simulink model "VB_RIFKF_UWB_INS25"  (R2023a)
settings: Solver=FixedStepAuto  StartTime=0.0  StopTime=500  FixedStep=0.01  RelTol=1e-3
InitFcn:
  | resilient_initNavigation1216;
  | init_param;
  | param_bias;
undefined symbols (not defined in the file or in its folder): dt, g0, gam0_rad, ISUS_flag, lp_GPS_sample_time, lp_Lidar_knoise, lp_Lidar_max, lp_Lidar_min, lp_Lidar_sample_time, lp_Lidar_seed, lp_UWB_knoise, lp_UWB_sample_time, lp_UWB_seed, lp_UWB_XY_max, lp_UWB_XY_min, magnitude, p, P0, P0_RIEKF, param, pd0, pe0, phi0_rad, pn0, psi, psi0_rad, state_dim, vd0, ve0, vn0
libraries: simulink_extras x108, simulink x89, dspstat3 x74, sharedtransform x61, matrix_library x11, sharedTrackingLibrary x8, aerolibconvert2 x5, aerolibtransform2 x5, dspfactors x3
(part 1 of 29)
settings Model: PacingRate=0.089000  Creator=Ye Xiaoyu  LastModifiedBy=18296
settings DataIOCC: SaveFormat=Structure
settings DebuggingCC: ParameterPrecisionLossMsg=none

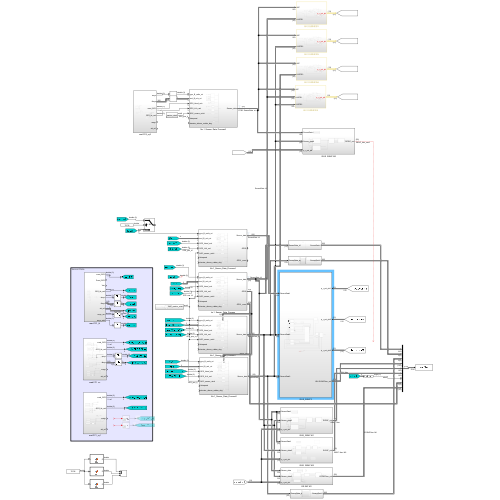
[thumbnail: Simulink's stored preview of the top-level diagram]
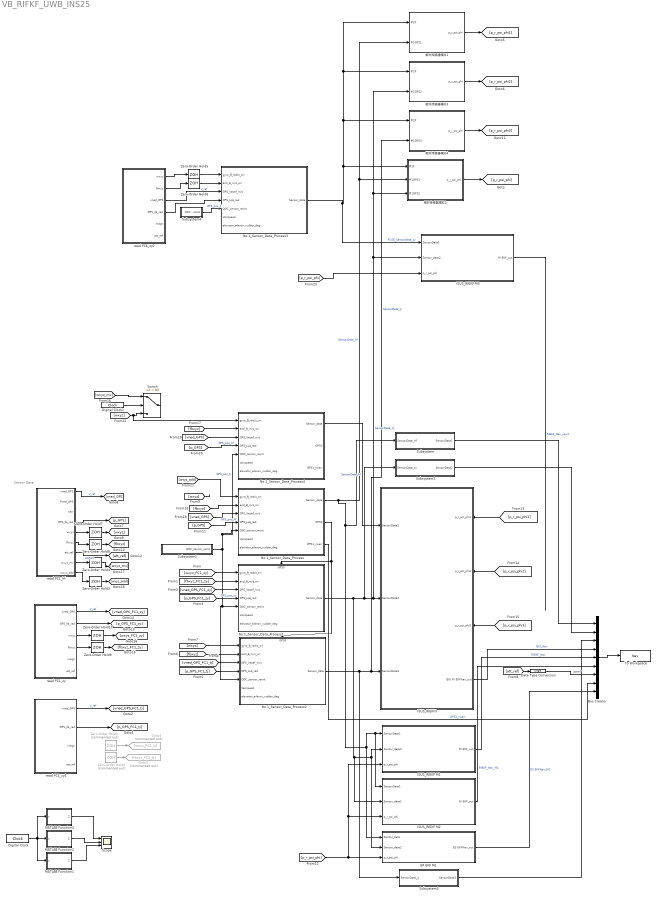
== system VB_RIFKF_UWB_INS25 ==
  note: Sensor Data
  Bus Creator : BusCreator  Inputs=9
  Data Type Conversion : DataTypeConversion  OutDataTypeStr=single  SaturateOnIntegerOverflow=off  RndMeth=Floor
  Digital Clock : DigitalClock  SampleTime=0.01
  Digital Clock1 : DigitalClock  SampleTime=0.01
  ER EKF M1 : Subsystem
  Goto3 : Goto  Commented=on  GotoTag=fbxyz_FC1_tj
  Goto4 : Goto  Commented=on  GotoTag=wxyz_FC1_tj
  ISUS_RIEKF M1 : Subsystem
  ISUS_RIEKF M2 : Subsystem
  ISUS_RIEKF M3 : Subsystem
  ISUS_RIEKF3 : Subsystem
      settings: PortSchema="{\"entries\":[{\"content\":{\"sides\":[{\"content\":{\"connectorIds\":[\"In1\",\"In2\",\"In3\"]},\"type\":\"ConnectorPlacement.EquallySpacedRectSide\",\"uuid\":\"2bcd161f-da55-4ee1-9ea8-951282ac87a0\"},{\"content\":{\"connectorIds\":[\"In4\",\"In5\",\"In6\",\"Out1\"],\"side\":\"RIGHT\"},\"type\":\"ConnectorPlacement.EquallySpacedRectSide\",\"uuid\":\"1132c6d7-5262-4ef0-a9d0-f977b200d157\"},{\"content\":{\"side\":\"TOP\"},\"type\":\"ConnectorPlacement.EquallySpacedRectSide\",\"uuid\":\"5bcb3a10-5be6-4cd2-9d61-0144f4936936\"}]},\"type\":\"ConnectorPlacement.EquallySpacedConnector\",\"uuid\":\"76638c5d-0c18-4b86-9384-f3a5e1322473\"}],\"packageUris\":[\"http://schema.mathworks.com/mf0/Connector/R2020b\"],\"version\":\"1.0\"}"
  MATLAB Function1 : MATLAB Function  TreatAsAtomicUnit=on
  MATLAB Function2 : MATLAB Function  TreatAsAtomicUnit=on
  MATLAB Function3 : MATLAB Function  TreatAsAtomicUnit=on
  No.1_Sensor_Data_Process : Subsystem
  No.1_Sensor_Data_Process1 : Subsystem
      settings: PortSchema="{\"entries\":[{\"content\":{\"sides\":[{\"content\":{\"connectorIds\":[\"In1\",\"In2\",\"In3\",\"In4\",\"In5\",\"In6\",\"In7\"]},\"type\":\"ConnectorPlacement.EquallySpacedRectSide\",\"uuid\":\"9a461442-5a4c-405b-8781-00f946dfe93c\"},{\"content\":{\"connectorIds\":[\"Out1\"],\"side\":\"RIGHT\"},\"type\":\"ConnectorPlacement.EquallySpacedRectSide\",\"uuid\":\"70ca8ff8-5980-4d24-aa39-0c8562a9d1d9\"},{\"content\":{\"connectorIds\":[\"In8\"],\"side\":\"TOP\"},\"type\":\"ConnectorPlacement.EquallySpacedRectSide\",\"uuid\":\"b1ebbd88-9925-4860-b235-fb3cc0770858\"}]},\"type\":\"ConnectorPlacement.EquallySpacedConnector\",\"uuid\":\"3dd6f087-9fad-422a-adf7-c884c798750f\"}],\"packageUris\":[\"http://schema.mathworks.com/mf0/Connector/R2020b\"],\"version\":\"1.0\"}"
  No.1_Sensor_Data_Process2 : Subsystem
      settings: PortSchema="{\"entries\":[{\"content\":{\"sides\":[{\"content\":{\"connectorIds\":[\"In1\",\"In2\",\"In3\",\"In4\",\"In5\",\"In6\",\"In7\"]},\"type\":\"ConnectorPlacement.EquallySpacedRectSide\",\"uuid\":\"9a461442-5a4c-405b-8781-00f946dfe93c\"},{\"content\":{\"connectorIds\":[\"Out1\"],\"side\":\"RIGHT\"},\"type\":\"ConnectorPlacement.EquallySpacedRectSide\",\"uuid\":\"70ca8ff8-5980-4d24-aa39-0c8562a9d1d9\"},{\"content\":{\"connectorIds\":[\"In8\"],\"side\":\"TOP\"},\"type\":\"ConnectorPlacement.EquallySpacedRectSide\",\"uuid\":\"b1ebbd88-9925-4860-b235-fb3cc0770858\"}]},\"type\":\"ConnectorPlacement.EquallySpacedConnector\",\"uuid\":\"3dd6f087-9fad-422a-adf7-c884c798750f\"}],\"packageUris\":[\"http://schema.mathworks.com/mf0/Connector/R2020b\"],\"version\":\"1.0\"}"
  No.1_Sensor_Data_Process3 : Subsystem
  No.1_Sensor_Data_Process4 : Subsystem
  Scope : Scope  NumInputPorts=3
  Subsystem : Subsystem
  Subsystem1 : Subsystem
  Subsystem2 : Subsystem
  Subsystem3 : Subsystem
  Subsystem4 : Subsystem
  Switch : Switch  Criteria=u2 > Threshold  Threshold=80  SaturateOnIntegerOverflow=off  InputSameDT=off
  To Workspace : ToWorkspace  VariableName=Nav  SaveFormat=Timeseries  SampleTime=0.01
  Zero-Order Hold1 : ZeroOrderHold  Commented=on  SampleTime=dt
  Zero-Order Hold{3..10} (8 alike) : ZeroOrderHold  SampleTime=dt
  Zero-Order Hold2 : ZeroOrderHold  Commented=on  SampleTime=dt
  read FC1_hf : Subsystem
  read FC1_zy : Subsystem
  read FC1_zy1 : Subsystem
  read FC6_zy2 : Subsystem
  相对传感器模拟1 : Subsystem
  相对传感器模拟2 : Subsystem
  相对传感器模拟3 : Subsystem
  相对传感器模拟4 : Subsystem
  wires:
  read FC1_hf/1(vned_GPS) -> [vned_GPS]  "V_ref"
  read FC1_hf/6(fbxyz) -> Zero-Order Hold8/1
  read FC1_hf/5(wxyz) -> Zero-Order Hold7/1
  read FC1_hf/7(att_ref) -> [att_ref]  "att_ref"
  read FC1_zy/2(GPS_lla_rad) -> [p_GPS_FC1_zy]
  read FC1_zy/1(vned_GPS) -> [vned_GPS_FC1_zy]  "V_ref"
  read FC1_hf/4(GPS_lla_rad) -> [p_GPS]
  Zero-Order Hold10/1 -> [wxyz_FC1_zy]
  Zero-Order Hold9/1 -> [fbxyz_FC1_zy]
  read FC1_zy/3(wxyz) -> Zero-Order Hold10/1
  read FC1_zy/4(fbxyz) -> Zero-Order Hold9/1
  Zero-Order Hold7/1 -> [wxyz]
  Zero-Order Hold8/1 -> [fbxyz]
  [fbxyz] -> No.1_Sensor_Data_Process/2(accl_B_m/s_ori)
  Subsystem1/1(QGC_sensor_reinit) -> No.1_Sensor_Data_Process4/5(QGC_sensor_reinit), No.1_Sensor_Data_Process/5(QGC_sensor_reinit), No.1_Sensor_Data_Process1/5(QGC_sensor_reinit), No.1_Sensor_Data_Process2/5(QGC_sensor_reinit)  "GPS_pos_tj"
  [wxyz] -> ?
  No.1_Sensor_Data_Process1/1(Sensor_data) -> ISUS_RIEKF3/2(SensorData2), 相对传感器模拟3/2(#1GPS2), 相对传感器模拟2/3(#1GPS2), ISUS_RIEKF M3/2(Sensor_data2), Subsystem2/1(SensorData_zy), ISUS_RIEKF M2/2(Sensor_data2), ER EKF M1/2(Sensor_data2), ISUS_RIEKF M1/2(Sensor_data2)  "SensorData_zy"
  [wxyz_FC1_zy] -> No.1_Sensor_Data_Process1/1(gyro_B_rad/s_ori)
  [fbxyz_FC1_zy] -> No.1_Sensor_Data_Process1/2(accl_B_m/s_ori)
  [vned_GPS] -> No.1_Sensor_Data_Process/3(GPS_Vecef_m/s)
  [p_GPS] -> No.1_Sensor_Data_Process/4(GPS_LLA_rad)  "GPS_pos_hf"
  [vned_GPS_FC1_zy] -> No.1_Sensor_Data_Process1/3(GPS_Vecef_m/s)
  [p_GPS_FC1_zy] -> No.1_Sensor_Data_Process1/4(GPS_LLA_rad)  "GPS_pos_zy"
  ? -> Zero-Order Hold2/1
  ? -> Zero-Order Hold1/1
  Zero-Order Hold2/1 -> Goto3/1
  Zero-Order Hold1/1 -> Goto4/1
  read FC1_zy1/1(vned_GPS) -> [vned_GPS_FC1_tj]  "V_ref"
  read FC1_zy1/2(GPS_lla_rad) -> [p_GPS_FC1_tj]
  [fbxyz] -> No.1_Sensor_Data_Process2/2(accl_B_m/s_ori)
  [wxyz] -> No.1_Sensor_Data_Process2/1(gyro_B_rad/s_ori)
  [vned_GPS_FC1_tj] -> No.1_Sensor_Data_Process2/3(GPS_Vecef_m/s)
  [p_GPS_FC1_tj] -> No.1_Sensor_Data_Process2/4(GPS_LLA_rad)
  No.1_Sensor_Data_Process2/1(Sensor_data) -> Subsystem3/1(SensorData_tj), ISUS_RIEKF3/3(SensorData3), 相对传感器模拟4/2(#1GPS3)  "SensorData_tj"
  ISUS_RIEKF3/1(ISIU RI EKFNav_out) -> Bus Creator/4  "ISIU_Nav"
  ISUS_RIEKF M1/1(RI EKF_out) -> Bus Creator/5  "RIEKF_Nav"
  Bus Creator/1 -> To Workspace/1
  Subsystem/1(SensorData1) -> Bus Creator/1
  Subsystem2/1(SensorData2) -> Bus Creator/2
  Subsystem3/1(SensorData3) -> Bus Creator/3
  [att_ref] -> Data Type Conversion/1
  Data Type Conversion/1 -> Bus Creator/7  "attref"
  No.1_Sensor_Data_Process/2(GPS0) -> No.1_Sensor_Data_Process2/8(GPS0), No.1_Sensor_Data_Process1/8(GPS0)
  No.1_Sensor_Data_Process/3(GPS1_noerr) -> Bus Creator/8  "GPS1_noerr"
  ISUS_RIEKF M2/1(RI EKF_out) -> Bus Creator/6  "RIEKF_Nav_M2"
  ER EKF M1/1(ES EKFNav_out) -> Bus Creator/9  "ES EKFNav_M1"
  Digital Clock/1 -> MATLAB Function3/1(t), MATLAB Function1/1(t), MATLAB Function2/1(t)
  MATLAB Function2/1(Z) -> Scope/2
  MATLAB Function1/1(Z) -> Scope/3
  MATLAB Function3/1(Z) -> Scope/1
  read FC6_zy2/4(GPS_lla_rad) -> No.1_Sensor_Data_Process3/4(GPS_LLA_rad)
  read FC6_zy2/3(vned_GPS) -> No.1_Sensor_Data_Process3/3(GPS_Vecef_m/s)  "V_ref"
  Subsystem4/1(QGC_sensor_reinit) -> No.1_Sensor_Data_Process3/5(QGC_sensor_reinit)  "GPS_pos_tj"
  No.1_Sensor_Data_Process3/1(Sensor_data) -> ISUS_RIEKF M3/1(SensorData1), 相对传感器模拟1/1(#2P), 相对传感器模拟3/1(#2P), 相对传感器模拟4/1(#2P), 相对传感器模拟2/1(#2P)  "FCS6_SensorData_zy"
  No.1_Sensor_Data_Process/1(Sensor_data) -> ER EKF M1/1(Sensor_data), ISUS_RIEKF M1/1(SensorData1), ISUS_RIEKF M2/1(SensorData1), Subsystem/1(SensorData_hf), 相对传感器模拟1/2(#1GPS1), 相对传感器模拟2/2(#1GPS1)  "SensorData_hf"
  相对传感器模拟2/1(p_r_psi_phi) -> [p_r_psi_phi]
  [p_r_psi_phi] -> ISUS_RIEKF M1/3(p_r_psi_phi), ISUS_RIEKF M2/3(p_r_psi_phi), ER EKF M1/3(p_r_psi_phi)
  相对传感器模拟1/1(p_r_psi_phi) -> [p_r_psi_phi1]
  相对传感器模拟3/1(p_r_psi_phi) -> [p_r_psi_phi2]
  相对传感器模拟4/1(p_r_psi_phi) -> [p_r_psi_phi3]
  [p_r_psi_phi1] -> ISUS_RIEKF3/4(p_r_psi_phi1)
  [p_r_psi_phi2] -> ISUS_RIEKF3/5(p_r_psi_phi2)
  [p_r_psi_phi3] -> ISUS_RIEKF3/6(p_r_psi_phi3)
  read FC1_hf/9(wxyz_add) -> Zero-Order Hold3/1
  read FC1_hf/8(wxyz_mv) -> Zero-Order Hold4/1
  Zero-Order Hold4/1 -> [wxyz_mv]
  Zero-Order Hold3/1 -> [wxyz_add]
  [wxyz_mv] -> Switch/1
  [fbxyz] -> No.1_Sensor_Data_Process4/2(accl_B_m/s_ori)
  [vned_GPS] -> No.1_Sensor_Data_Process4/3(GPS_Vecef_m/s)
  [p_GPS] -> No.1_Sensor_Data_Process4/4(GPS_LLA_rad)  "GPS_pos_hf"
  No.1_Sensor_Data_Process4/1(Sensor_data) -> ISUS_RIEKF3/1(SensorData1)  "SensorData_hf"
  [wxyz_add] -> No.1_Sensor_Data_Process/1(gyro_B_rad/s_ori)
  Digital Clock1/1 -> Switch/2
  [wxyz] -> No.1_Sensor_Data_Process4/1(gyro_B_rad/s_ori), Switch/3
  [p_r_psi_phi] -> ISUS_RIEKF M3/3(p_r_psi_phi)
  ISUS_RIEKF M3/1(RI EKF_out) -> ?  "RIEKF_Nav_uav2"
  read FC6_zy2/2(fbxyz) -> Zero-Order Hold6/1
  read FC6_zy2/1(wxyz) -> Zero-Order Hold5/1
  Zero-Order Hold5/1 -> No.1_Sensor_Data_Process3/1(gyro_B_rad/s_ori)
  Zero-Order Hold6/1 -> No.1_Sensor_Data_Process3/2(accl_B_m/s_ori)

== system VB_RIFKF_UWB_INS25/ER EKF M1 ==
  Sensor_data : Inport
  Sensor_data2 : Inport  Port=2
  p_r_psi_phi : Inport  Port=3
  Bus_Constructor : Subsystem
  Bus_Constructor2 : Subsystem
  Data Store Memory : DataStoreMemory  DataStoreName=feedback_flag_18dim  WriteAfterWriteMsg=warning  ShowAdditionalParam=off
  Data Store Memory1 : DataStoreMemory  DataStoreName=GPS_enable  WriteAfterWriteMsg=warning  ShowAdditionalParam=off
  Data Store Read : DataStoreRead  DataStoreName=GPS_enable  IndexOptions=Index vector (dialog)  Indices=1  OutputSizes=1
  Error State Kalman Filter : Subsystem
  INS propogation : Subsystem
  Sensor_data1 : InportShadow
  ES EKFNav_out : Outport
  wires:
  Sensor_data/1 -> INS propogation/1(Sensor_data)
  Error State Kalman Filter/1(delta_state) -> INS propogation/3(delta_state)
  Error State Kalman Filter/2(Measuemrnt Enable Flag) -> INS propogation/2(Measuemrnt Enable Flag)
  INS propogation/1(INSstate) -> Bus_Constructor/1(INSstate), Error State Kalman Filter/2(INS state)
  Sensor_data1/1 -> Error State Kalman Filter/1(Sensor_data)
  Bus_Constructor/1(TranslationData) -> Bus_Constructor2/1(TranlationData)
  Bus_Constructor/2(RotationData) -> Bus_Constructor2/2(RotationData)
  Bus_Constructor/3(INSbiasData) -> Bus_Constructor2/3(INSbiasData)
  Bus_Constructor2/1(RI EKFNav_out) -> ES EKFNav_out/1  "RI EKF_out"
  Sensor_data2/1 -> Error State Kalman Filter/3(Sensor_data2)
  p_r_psi_phi/1 -> Error State Kalman Filter/4(p_r_psi_phi)

== system VB_RIFKF_UWB_INS25/ISUS_RIEKF M1 ==
  SensorData1 : Inport
  Sensor_data2 : Inport  Port=2
  p_r_psi_phi : Inport  Port=3
  Bus Selector : BusSelector  OutputSignals=delta_state
  Bus_Constructor : Subsystem
  Bus_Constructor2 : Subsystem
  Data Store Memory : DataStoreMemory  DataStoreName=feedback_flag_18dim_RIEKF  WriteAfterWriteMsg=warning  ShowAdditionalParam=off
  Data Store Memory1 : DataStoreMemory  DataStoreName=GPS_enable_RIEKF  WriteAfterWriteMsg=warning  ShowAdditionalParam=off
  Error State Kalman Filter M1 : Subsystem
      settings: PortSchema="{\"entries\":[{\"content\":{\"sides\":[{\"content\":{\"connectorIds\":[\"In1\",\"In2\"]},\"type\":\"ConnectorPlacement.EquallySpacedRectSide\",\"uuid\":\"06174571-c694-4df4-9d5d-6f87fae6fca4\"},{\"content\":{\"connectorIds\":[\"Out1\",\"In3\",\"Out2\",\"In4\"],\"side\":\"RIGHT\"},\"type\":\"ConnectorPlacement.EquallySpacedRectSide\",\"uuid\":\"968b9d6c-6269-4201-a494-e936bbf59a60\"},{\"content\":{\"side\":\"TOP\"},\"type\":\"ConnectorPlacement.EquallySpacedRectSide\",\"uuid\":\"42ff394f-5689-4ff8-9152-3bae82104e67\"}]},\"type\":\"ConnectorPlacement.EquallySpacedConnector\",\"uuid\":\"445a129c-1b79-435d-8e29-ecc9e3655f53\"}],\"packageUris\":[\"http://schema.mathworks.com/mf0/Connector/R2020b\"],\"version\":\"1.0\"}"
  INS propogation : Subsystem
  Sensor_data1 : InportShadow
  RI EKF_out : Outport
  wires:
  Bus_Constructor2/1(RI EKFNav_out) -> RI EKF_out/1  "RI EKF_out"
  Bus_Constructor/4(GNSS enable flag) -> Bus_Constructor2/4(GNSS enable flag)
  Bus_Constructor/3(INSbiasData) -> Bus_Constructor2/3(INSbiasData)  "INSbiasData"
  Bus_Constructor/2(RotationData) -> Bus_Constructor2/2(RotationData)  "RotationData"
  Bus_Constructor/1(TranslationData) -> Bus_Constructor2/1(TranlationData)  "TranslationData"
  Error State Kalman Filter M1/2(EKFstate_M1) -> Bus Selector/1
  SensorData1/1 -> INS propogation/1(Sensor_data)
  Error State Kalman Filter M1/1(Measuemrnt Enable Flag) -> INS propogation/2(Measuemrnt Enable Flag)
  INS propogation/1(INSstate) -> Bus_Constructor/1(INSstate), Error State Kalman Filter M1/2(INS state)
  Sensor_data1/1 -> Error State Kalman Filter M1/1(Sensor_data)
  Bus Selector/1 -> INS propogation/3(delta_state)  "<delta_state>"
  Sensor_data2/1 -> Error State Kalman Filter M1/3(Sensor_data2)
  p_r_psi_phi/1 -> Error State Kalman Filter M1/4(p_r_psi_phi1)

== system VB_RIFKF_UWB_INS25/ISUS_RIEKF M2 ==
  SensorData1 : Inport
  Sensor_data2 : Inport  Port=2
  p_r_psi_phi : Inport  Port=3
  Bus Selector : BusSelector  OutputSignals=delta_state
  Bus_Constructor : Subsystem
  Bus_Constructor2 : Subsystem
  Data Store Memory : DataStoreMemory  DataStoreName=feedback_flag_18dim_RIEKF  WriteAfterWriteMsg=warning  ShowAdditionalParam=off
  Data Store Memory1 : DataStoreMemory  DataStoreName=GPS_enable_RIEKF  WriteAfterWriteMsg=warning  ShowAdditionalParam=off
  Error State Kalman Filter M1 : Subsystem
      settings: PortSchema="{\"entries\":[{\"content\":{\"sides\":[{\"content\":{\"connectorIds\":[\"In1\",\"In2\"]},\"type\":\"ConnectorPlacement.EquallySpacedRectSide\",\"uuid\":\"06174571-c694-4df4-9d5d-6f87fae6fca4\"},{\"content\":{\"connectorIds\":[\"Out1\",\"In3\",\"Out2\",\"In4\"],\"side\":\"RIGHT\"},\"type\":\"ConnectorPlacement.EquallySpacedRectSide\",\"uuid\":\"968b9d6c-6269-4201-a494-e936bbf59a60\"},{\"content\":{\"side\":\"TOP\"},\"type\":\"ConnectorPlacement.EquallySpacedRectSide\",\"uuid\":\"42ff394f-5689-4ff8-9152-3bae82104e67\"}]},\"type\":\"ConnectorPlacement.EquallySpacedConnector\",\"uuid\":\"445a129c-1b79-435d-8e29-ecc9e3655f53\"}],\"packageUris\":[\"http://schema.mathworks.com/mf0/Connector/R2020b\"],\"version\":\"1.0\"}"
  Error State Kalman Filter M3 : Subsystem  Commented=on
  Error State Kalman Filter M4 : Subsystem  Commented=on
      settings: PortSchema="{\"entries\":[{\"content\":{\"sides\":[{\"content\":{\"connectorIds\":[\"In1\",\"In2\"]},\"type\":\"ConnectorPlacement.EquallySpacedRectSide\",\"uuid\":\"06174571-c694-4df4-9d5d-6f87fae6fca4\"},{\"content\":{\"connectorIds\":[\"Out1\",\"In3\",\"Out2\",\"In4\"],\"side\":\"RIGHT\"},\"type\":\"ConnectorPlacement.EquallySpacedRectSide\",\"uuid\":\"968b9d6c-6269-4201-a494-e936bbf59a60\"},{\"content\":{\"side\":\"TOP\"},\"type\":\"ConnectorPlacement.EquallySpacedRectSide\",\"uuid\":\"42ff394f-5689-4ff8-9152-3bae82104e67\"}]},\"type\":\"ConnectorPlacement.EquallySpacedConnector\",\"uuid\":\"445a129c-1b79-435d-8e29-ecc9e3655f53\"}],\"packageUris\":[\"http://schema.mathworks.com/mf0/Connector/R2020b\"],\"version\":\"1.0\"}"
  INS propogation1 : Subsystem
  INS propogation2 : Subsystem  Commented=on
  Sensor_data1 : InportShadow
  RI EKF_out : Outport
  wires:
  Bus Selector/1 -> INS propogation1/3(delta_state)  "<delta_state>"
  Sensor_data1/1 -> Error State Kalman Filter M1/1(Sensor_data)
  INS propogation1/1(INSstate) -> Error State Kalman Filter M1/2(INS state), Bus_Constructor/1(INSstate)
  SensorData1/1 -> INS propogation1/1(Sensor_data)
  Error State Kalman Filter M1/2(EKFstate_M1) -> Bus Selector/1
  Bus_Constructor/1(TranslationData) -> Bus_Constructor2/1(TranlationData)  "TranslationData"
  Bus_Constructor/2(RotationData) -> Bus_Constructor2/2(RotationData)  "RotationData"
  Bus_Constructor/3(INSbiasData) -> Bus_Constructor2/3(INSbiasData)  "INSbiasData"
  Bus_Constructor/4(GNSS enable flag) -> Bus_Constructor2/4(GNSS enable flag)
  Bus_Constructor2/1(RI EKFNav_out) -> RI EKF_out/1  "RI EKF_out"
  Error State Kalman Filter M1/1(Measuemrnt Enable Flag) -> INS propogation1/2(Measuemrnt Enable Flag)
  Sensor_data2/1 -> Error State Kalman Filter M1/3(Sensor_data2)
  p_r_psi_phi/1 -> Error State Kalman Filter M1/4(p_r_psi_phi1)

== system VB_RIFKF_UWB_INS25/ISUS_RIEKF M3 ==
  SensorData1 : Inport
  Sensor_data2 : Inport  Port=2
  p_r_psi_phi : Inport  Port=3
  Bus Selector : BusSelector  OutputSignals=delta_state
  Bus_Constructor : Subsystem
  Bus_Constructor2 : Subsystem
  Data Store Memory : DataStoreMemory  DataStoreName=feedback_flag_18dim_RIEKF  WriteAfterWriteMsg=warning  ShowAdditionalParam=off
  Data Store Memory1 : DataStoreMemory  DataStoreName=GPS_enable_RIEKF  WriteAfterWriteMsg=warning  ShowAdditionalParam=off
  Error State Kalman Filter M1 : Subsystem
      settings: PortSchema="{\"entries\":[{\"content\":{\"sides\":[{\"content\":{\"connectorIds\":[\"In1\",\"In2\"]},\"type\":\"ConnectorPlacement.EquallySpacedRectSide\",\"uuid\":\"06174571-c694-4df4-9d5d-6f87fae6fca4\"},{\"content\":{\"connectorIds\":[\"Out1\",\"In3\",\"Out2\",\"In4\"],\"side\":\"RIGHT\"},\"type\":\"ConnectorPlacement.EquallySpacedRectSide\",\"uuid\":\"968b9d6c-6269-4201-a494-e936bbf59a60\"},{\"content\":{\"side\":\"TOP\"},\"type\":\"ConnectorPlacement.EquallySpacedRectSide\",\"uuid\":\"42ff394f-5689-4ff8-9152-3bae82104e67\"}]},\"type\":\"ConnectorPlacement.EquallySpacedConnector\",\"uuid\":\"445a129c-1b79-435d-8e29-ecc9e3655f53\"}],\"packageUris\":[\"http://schema.mathworks.com/mf0/Connector/R2020b\"],\"version\":\"1.0\"}"
  INS propogation : Subsystem
  Sensor_data1 : InportShadow
  RI EKF_out : Outport
  wires:
  Bus_Constructor2/1(RI EKFNav_out) -> RI EKF_out/1  "RI EKF_out"
  Bus_Constructor/4(GNSS enable flag) -> Bus_Constructor2/4(GNSS enable flag)
  Bus_Constructor/3(INSbiasData) -> Bus_Constructor2/3(INSbiasData)  "INSbiasData"
  Bus_Constructor/2(RotationData) -> Bus_Constructor2/2(RotationData)  "RotationData"
  Bus_Constructor/1(TranslationData) -> Bus_Constructor2/1(TranlationData)  "TranslationData"
  Error State Kalman Filter M1/2(EKFstate_M1) -> Bus Selector/1
  SensorData1/1 -> INS propogation/1(Sensor_data)
  Error State Kalman Filter M1/1(Measuemrnt Enable Flag) -> INS propogation/2(Measuemrnt Enable Flag)
  INS propogation/1(INSstate) -> Bus_Constructor/1(INSstate), Error State Kalman Filter M1/2(INS state)
  Sensor_data1/1 -> Error State Kalman Filter M1/1(Sensor_data)
  Bus Selector/1 -> INS propogation/3(delta_state)  "<delta_state>"
  Sensor_data2/1 -> Error State Kalman Filter M1/3(Sensor_data2)
  p_r_psi_phi/1 -> Error State Kalman Filter M1/4(p_r_psi_phi1)

== system VB_RIFKF_UWB_INS25/ISUS_RIEKF3 ==
  SensorData1 : Inport
  SensorData2 : Inport  Port=2
  SensorData3 : Inport  Port=3
  p_r_psi_phi1 : Inport  Port=4
  p_r_psi_phi2 : Inport  Port=5
  p_r_psi_phi3 : Inport  Port=6
  Bus Creator : BusCreator  Inputs=2
  Bus_Constructor : Subsystem
  Bus_Constructor2 : Subsystem
      settings: PortSchema="{\"entries\":[{\"content\":{\"sides\":[{\"content\":{\"connectorIds\":[\"In1\",\"In2\",\"In3\",\"In4\",\"In5\",\"In6\",\"In7\"]},\"type\":\"ConnectorPlacement.EquallySpacedRectSide\",\"uuid\":\"2ada5c99-a5a9-492d-97a7-10d7c05175d7\"},{\"content\":{\"connectorIds\":[\"Out1\"],\"side\":\"RIGHT\"},\"type\":\"ConnectorPlacement.EquallySpacedRectSide\",\"uuid\":\"cde580e4-aba0-41e6-ab1b-1e880cd106da\"},{\"content\":{\"side\":\"TOP\"},\"type\":\"ConnectorPlacement.EquallySpacedRectSide\",\"uuid\":\"542037bf-a2f3-4431-b2f0-0d887f8b5219\"},{\"content\":{\"connectorIds\":[\"In8\"],\"side\":\"BOTTOM\"},\"type\":\"ConnectorPlacement.EquallySpacedRectSide\",\"uuid\":\"59daa5b1-1426-4f22-83e7-df6003f21326\"}]},\"type\":\"ConnectorPlacement.EquallySpacedConnector\",\"uuid\":\"47431650-46c1-4f35-bd73-f1f710c66ac0\"}],\"packageUris\":[\"http://schema.mathworks.com/mf0/Connector/R2020b\"],\"version\":\"1.0\"}"
  Data Store Memory : DataStoreMemory  DataStoreName=feedback_flag_18dim_RIEKF  WriteAfterWriteMsg=warning  ShowAdditionalParam=off
  Data Store Memory1 : DataStoreMemory  DataStoreName=GPS_enable_RIEKF  WriteAfterWriteMsg=warning  ShowAdditionalParam=off
  Error State Kalman Filter M1 : Subsystem
  Error State Kalman Filter M2 : Subsystem
  Error State Kalman Filter M4 : Subsystem
  Extract Diagonal1 : matrix_library/Extract Diagonal
  INS propogation : Subsystem
  INS propogation1 : Subsystem
  INS propogation2 : Subsystem
  INS propogation3 : Subsystem
  Reshape : Reshape
  Scope2 : Scope
  Sensor_data1 : InportShadow
  Subsystem : Subsystem
  Terminator : Terminator
  Terminator2 : Terminator
  ISIU RI EKFNav_out : Outport
  wires:
  Extract Diagonal1/1 -> Scope2/1  "covariance_diag"
  Subsystem/1(P_mixed_RIEKF_M1) -> Error State Kalman Filter M4/3(P_mixed_RIEKF_model1)
  Reshape/1 -> Bus Creator/2
  Bus Creator/1 -> Bus_Constructor2/8(ISIU)
  ? -> Reshape/1  "L_k"
  ? -> Bus Creator/1  "mu_k"
  Subsystem/7(X_mixed_RIEKF_M3) -> Error State Kalman Filter M2/4(X_mixed_RIEKF_M3)
  Subsystem/8(P_mixed_RIEKF_M3) -> Error State Kalman Filter M2/3(P_mixed_RIEKF_model3)
  Error State Kalman Filter M2/2(EKFstate_M3) -> Bus_Constructor2/7(EKFstate_M3), Subsystem/3(EKFstate_M3)
  Error State Kalman Filter M2/1(Measuemrnt Enable Flag) -> Terminator2/1
  SensorData3/1 -> Error State Kalman Filter M2/1(Sensor_data)
  Subsystem/6(pk_k) -> Extract Diagonal1/1
  Bus_Constructor2/1(RI EKFNav_out) -> ISIU RI EKFNav_out/1  "ISIU RI EKFNav_out"
  Bus_Constructor/4(GNSS enable flag) -> Bus_Constructor2/4(GNSS enable flag)
  Bus_Constructor/3(INSbiasData) -> Bus_Constructor2/3(INSbiasData)  "INSbiasData"
  Bus_Constructor/2(RotationData) -> Bus_Constructor2/2(RotationData)  "RotationData"
  Bus_Constructor/1(TranslationData) -> Bus_Constructor2/1(TranlationData)  "TranslationData"
  Error State Kalman Filter M4/2(EKFstate_M1) -> Bus_Constructor2/5(EKFstate_M1), Subsystem/1(EKFstate_M1)
  Subsystem/4(X_mixed_RIEKF_M2) -> Error State Kalman Filter M1/4(X_mixed_RIEKF_M2)
  Subsystem/3(P_mixed_RIEKF_M2) -> Error State Kalman Filter M1/3(P_mixed_RIEKF_model2)
  Subsystem/2(X_mixed_RIEKF_M1) -> Error State Kalman Filter M4/4(X_mixed_RIEKF_M1)
  Error State Kalman Filter M1/2(EKFstate_M2) -> Bus_Constructor2/6(EKFstate_M2), Subsystem/2(EKFstate_M2)
  Error State Kalman Filter M1/1(Measuemrnt Enable Flag) -> Terminator/1
  SensorData2/1 -> Error State Kalman Filter M1/1(Sensor_data)
  SensorData1/1 -> INS propogation/1(Sensor_data), INS propogation1/1(Sensor_data), INS propogation2/1(Sensor_data), INS propogation3/1(Sensor_data)
  Error State Kalman Filter M4/1(Measuemrnt Enable Flag) -> INS propogation3/2(Measuemrnt Enable Flag), INS propogation2/2(Measuemrnt Enable Flag), INS propogation1/2(Measuemrnt Enable Flag), INS propogation/2(Measuemrnt Enable Flag)
  Sensor_data1/1 -> Error State Kalman Filter M4/1(Sensor_data)
  Error State Kalman Filter M4/3(delta_state) -> INS propogation1/3(delta_state)
  Error State Kalman Filter M2/3(delta_state) -> INS propogation3/3(delta_state)
  Subsystem/5(xk_k) -> INS propogation/3(delta_state)
  INS propogation/1(INSstate) -> Bus_Constructor/1(INSstate)
  Error State Kalman Filter M1/3(delta_state) -> INS propogation2/3(delta_state)
  INS propogation2/1(INSstate) -> Error State Kalman Filter M1/2(INS state)
  INS propogation3/1(INSstate) -> Error State Kalman Filter M2/2(INS state)
  INS propogation1/1(INSstate) -> Error State Kalman Filter M4/2(INS state)
  p_r_psi_phi1/1 -> Error State Kalman Filter M4/5(p_r_psi_phi1)
  p_r_psi_phi2/1 -> Error State Kalman Filter M1/5(p_r_psi_phi2)
  p_r_psi_phi3/1 -> Error State Kalman Filter M2/5(p_r_psi_phi3)

== system VB_RIFKF_UWB_INS25/No.1_Sensor_Data_Process ==
  gyro_B_rad/s_ori : Inport
  accl_B_m/s_ori : Inport  Port=2
  GPS_Vecef_m/s : Inport  Port=3
  GPS_LLA_rad : Inport  Port=4
  QGC_sensor_reinit : Inport  Port=5
  Vairspeed : Inport  Port=6
  elevator_aileron_rudder_deg : Inport  Port=7
  Bus Creator : BusCreator  Inputs=8
  Constant3 : Constant
  Constant4 : Constant  Value=0.8
  Data Type Conversion{,1..3,5..6,8..11} (10 alike) : DataTypeConversion  OutDataTypeStr=single  SaturateOnIntegerOverflow=off  RndMeth=Floor
  Data Type Conversion4 : DataTypeConversion  OutDataTypeStr=uint8  SaturateOnIntegerOverflow=off  RndMeth=Floor
  Data Type Conversion7 : DataTypeConversion  OutDataTypeStr=double  SaturateOnIntegerOverflow=off  RndMeth=Floor
  GPS_Data_Process : Subsystem
  IMU_Data_Process : Subsystem
  Magn_Data_Process : Subsystem
  Mux : Mux  Inputs=3
  QGC_sensor_reinit1 : InportShadow  Port=5
  QGC_sensor_reinit2 : InportShadow  Port=5
  Subsystem : Subsystem
  TOF_Data_Process : Subsystem
  baro_Data_Process : Subsystem
  Sensor_data : Outport
  GPS0 : Outport  Port=2
  GPS1_noerr : Outport  Port=3
  wires:
  QGC_sensor_reinit2/1 -> TOF_Data_Process/2(QGC_sensor_reinit)  "QGC_sensor_reinit"
  Data Type Conversion3/1 -> baro_Data_Process/3(baro_tem)
  Data Type Conversion10/1 -> TOF_Data_Process/1(TOF_mm_ori)
  Data Type Conversion6/1 -> Magn_Data_Process/1(magn_B_guass_ori)
  Data Type Conversion5/1 -> baro_Data_Process/1(baro)
  Data Type Conversion9/1 -> GPS_Data_Process/4(hdop_GPS)
  Data Type Conversion4/1 -> GPS_Data_Process/3(GPS_fixtype)
  Data Type Conversion7/1 -> GPS_Data_Process/2(GPS_LLA_rad)
  Data Type Conversion2/1 -> GPS_Data_Process/1(GPS_Vecef_m/s)
  Data Type Conversion1/1 -> IMU_Data_Process/2(accl_B_m/s_ori)
  Data Type Conversion/1 -> IMU_Data_Process/1(gyro_B_rad/s_ori)
  TOF_Data_Process/1(TOF_Data) -> Bus Creator/5
  QGC_sensor_reinit1/1 -> Bus Creator/7  "QGC_sensor_reinit"
  Bus Creator/1 -> Sensor_data/1
  GPS_Vecef_m/s/1 -> Data Type Conversion2/1
  GPS_LLA_rad/1 -> Data Type Conversion7/1
  accl_B_m/s_ori/1 -> Data Type Conversion1/1
  Magn_Data_Process/1(MAGN_Data) -> Bus Creator/4  "MAGN_Data"
  gyro_B_rad/s_ori/1 -> Data Type Conversion/1
  baro_Data_Process/1(BARO_Data) -> Bus Creator/3  "BARO_Data"
  IMU_Data_Process/1(IMU_Data) -> Bus Creator/1  "IMU_Data"
  GPS_Data_Process/1(GPS_Data) -> Bus Creator/2  "GPS_Data"
  QGC_sensor_reinit/1 -> GPS_Data_Process/5(QGC_sensor_reinit), baro_Data_Process/2(QGC_sensor_reinit)  "QGC_sensor_reinit"
  Vairspeed/1 -> Data Type Conversion8/1  "VairspeedData"
  Data Type Conversion8/1 -> Subsystem/1(Vairspeed)
  Subsystem/1(VairspeedData) -> Bus Creator/6
  elevator_aileron_rudder_deg/1 -> Data Type Conversion11/1  "elevator_aileron_rudder_deg"
  Data Type Conversion11/1 -> Bus Creator/8  "elevator_aileron_rudder_deg"
  Constant3/1 -> Data Type Conversion4/1
  Constant4/1 -> Data Type Conversion9/1
  Mux/1 -> Data Type Conversion6/1
  GPS_Data_Process/2(GPS0) -> GPS0/1
  GPS_Data_Process/3(GPS_noerr) -> GPS1_noerr/1

== system VB_RIFKF_UWB_INS25/No.1_Sensor_Data_Process1 ==
  gyro_B_rad/s_ori : Inport
  accl_B_m/s_ori : Inport  Port=2
  GPS_Vecef_m/s : Inport  Port=3
  GPS_LLA_rad : Inport  Port=4
  QGC_sensor_reinit : Inport  Port=5
  Vairspeed : Inport  Port=6
  elevator_aileron_rudder_deg : Inport  Port=7
  GPS0 : Inport  Port=8
  Bus Creator : BusCreator  Inputs=8
  Constant3 : Constant
  Constant4 : Constant  Value=0.8
  Data Type Conversion{,1..3,5..6,8..11} (10 alike) : DataTypeConversion  OutDataTypeStr=single  SaturateOnIntegerOverflow=off  RndMeth=Floor
  Data Type Conversion4 : DataTypeConversion  OutDataTypeStr=uint8  SaturateOnIntegerOverflow=off  RndMeth=Floor
  Data Type Conversion7 : DataTypeConversion  OutDataTypeStr=double  SaturateOnIntegerOverflow=off  RndMeth=Floor
  GPS_Data_Process : Subsystem
  IMU_Data_Process : Subsystem
  Magn_Data_Process : Subsystem
  Mux : Mux  Inputs=3
  QGC_sensor_reinit1 : InportShadow  Port=5
  QGC_sensor_reinit2 : InportShadow  Port=5
  Subsystem : Subsystem
  TOF_Data_Process : Subsystem
  baro_Data_Process : Subsystem
  Sensor_data : Outport
  wires:
  Mux/1 -> Data Type Conversion6/1
  Constant4/1 -> Data Type Conversion9/1
  Constant3/1 -> Data Type Conversion4/1
  Data Type Conversion11/1 -> Bus Creator/8  "elevator_aileron_rudder_deg"
  elevator_aileron_rudder_deg/1 -> Data Type Conversion11/1  "elevator_aileron_rudder_deg"
  Subsystem/1(VairspeedData) -> Bus Creator/6
  Data Type Conversion8/1 -> Subsystem/1(Vairspeed)
  Vairspeed/1 -> Data Type Conversion8/1  "VairspeedData"
  QGC_sensor_reinit/1 -> baro_Data_Process/2(QGC_sensor_reinit), GPS_Data_Process/5(QGC_sensor_reinit)  "QGC_sensor_reinit"
  GPS_Data_Process/1(GPS_Data) -> Bus Creator/2  "GPS_Data"
  IMU_Data_Process/1(IMU_Data) -> Bus Creator/1  "IMU_Data"
  baro_Data_Process/1(BARO_Data) -> Bus Creator/3  "BARO_Data"
  gyro_B_rad/s_ori/1 -> Data Type Conversion/1
  Magn_Data_Process/1(MAGN_Data) -> Bus Creator/4  "MAGN_Data"
  accl_B_m/s_ori/1 -> Data Type Conversion1/1
  GPS_LLA_rad/1 -> Data Type Conversion7/1
  GPS_Vecef_m/s/1 -> Data Type Conversion2/1
  Bus Creator/1 -> Sensor_data/1
  QGC_sensor_reinit1/1 -> Bus Creator/7  "QGC_sensor_reinit"
  TOF_Data_Process/1(TOF_Data) -> Bus Creator/5
  Data Type Conversion/1 -> IMU_Data_Process/1(gyro_B_rad/s_ori)
  Data Type Conversion1/1 -> IMU_Data_Process/2(accl_B_m/s_ori)
  Data Type Conversion2/1 -> GPS_Data_Process/1(GPS_Vecef_m/s)
  Data Type Conversion7/1 -> GPS_Data_Process/2(GPS_LLA_rad)
  Data Type Conversion4/1 -> GPS_Data_Process/3(GPS_fixtype)
  Data Type Conversion9/1 -> GPS_Data_Process/4(hdop_GPS)
  Data Type Conversion5/1 -> baro_Data_Process/1(baro)
  Data Type Conversion6/1 -> Magn_Data_Process/1(magn_B_guass_ori)
  Data Type Conversion10/1 -> TOF_Data_Process/1(TOF_mm_ori)
  Data Type Conversion3/1 -> baro_Data_Process/3(baro_tem)
  QGC_sensor_reinit2/1 -> TOF_Data_Process/2(QGC_sensor_reinit)  "QGC_sensor_reinit"
  GPS0/1 -> GPS_Data_Process/6(GPS0)

== system VB_RIFKF_UWB_INS25/No.1_Sensor_Data_Process2 ==
  gyro_B_rad/s_ori : Inport
  accl_B_m/s_ori : Inport  Port=2
  GPS_Vecef_m/s : Inport  Port=3
  GPS_LLA_rad : Inport  Port=4
  QGC_sensor_reinit : Inport  Port=5
  Vairspeed : Inport  Port=6
  elevator_aileron_rudder_deg : Inport  Port=7
  GPS0 : Inport  Port=8
  Bus Creator : BusCreator  Inputs=8
  Constant3 : Constant
  Constant4 : Constant  Value=0.8
  Data Type Conversion{,1..3,5..6,8..11} (10 alike) : DataTypeConversion  OutDataTypeStr=single  SaturateOnIntegerOverflow=off  RndMeth=Floor
  Data Type Conversion4 : DataTypeConversion  OutDataTypeStr=uint8  SaturateOnIntegerOverflow=off  RndMeth=Floor
  Data Type Conversion7 : DataTypeConversion  OutDataTypeStr=double  SaturateOnIntegerOverflow=off  RndMeth=Floor
  GPS_Data_Process : Subsystem
  IMU_Data_Process : Subsystem
  Magn_Data_Process : Subsystem
  Mux : Mux  Inputs=3
  QGC_sensor_reinit1 : InportShadow  Port=5
  QGC_sensor_reinit2 : InportShadow  Port=5
  Subsystem : Subsystem
  TOF_Data_Process : Subsystem
  baro_Data_Process : Subsystem
  Sensor_data : Outport
  wires:
  QGC_sensor_reinit2/1 -> TOF_Data_Process/2(QGC_sensor_reinit)  "QGC_sensor_reinit"
  Data Type Conversion3/1 -> baro_Data_Process/3(baro_tem)
  Data Type Conversion10/1 -> TOF_Data_Process/1(TOF_mm_ori)
  Data Type Conversion6/1 -> Magn_Data_Process/1(magn_B_guass_ori)
  Data Type Conversion5/1 -> baro_Data_Process/1(baro)
  Data Type Conversion9/1 -> GPS_Data_Process/4(hdop_GPS)
  Data Type Conversion4/1 -> GPS_Data_Process/3(GPS_fixtype)
  Data Type Conversion7/1 -> GPS_Data_Process/2(GPS_LLA_rad)
  Data Type Conversion2/1 -> GPS_Data_Process/1(GPS_Vecef_m/s)
  Data Type Conversion1/1 -> IMU_Data_Process/2(accl_B_m/s_ori)
  Data Type Conversion/1 -> IMU_Data_Process/1(gyro_B_rad/s_ori)
  TOF_Data_Process/1(TOF_Data) -> Bus Creator/5
  QGC_sensor_reinit1/1 -> Bus Creator/7  "QGC_sensor_reinit"
  Bus Creator/1 -> Sensor_data/1
  GPS_Vecef_m/s/1 -> Data Type Conversion2/1
  GPS_LLA_rad/1 -> Data Type Conversion7/1
  accl_B_m/s_ori/1 -> Data Type Conversion1/1
  Magn_Data_Process/1(MAGN_Data) -> Bus Creator/4  "MAGN_Data"
  gyro_B_rad/s_ori/1 -> Data Type Conversion/1
  baro_Data_Process/1(BARO_Data) -> Bus Creator/3  "BARO_Data"
  IMU_Data_Process/1(IMU_Data) -> Bus Creator/1  "IMU_Data"
  GPS_Data_Process/1(GPS_Data) -> Bus Creator/2  "GPS_Data"
  QGC_sensor_reinit/1 -> GPS_Data_Process/5(QGC_sensor_reinit), baro_Data_Process/2(QGC_sensor_reinit)  "QGC_sensor_reinit"
  Vairspeed/1 -> Data Type Conversion8/1  "VairspeedData"
  Data Type Conversion8/1 -> Subsystem/1(Vairspeed)
  Subsystem/1(VairspeedData) -> Bus Creator/6
  elevator_aileron_rudder_deg/1 -> Data Type Conversion11/1  "elevator_aileron_rudder_deg"
  Data Type Conversion11/1 -> Bus Creator/8  "elevator_aileron_rudder_deg"
  Constant3/1 -> Data Type Conversion4/1
  Constant4/1 -> Data Type Conversion9/1
  Mux/1 -> Data Type Conversion6/1
  GPS0/1 -> GPS_Data_Process/6(GPS0)

== system VB_RIFKF_UWB_INS25/No.1_Sensor_Data_Process3 ==
  gyro_B_rad/s_ori : Inport
  accl_B_m/s_ori : Inport  Port=2
  GPS_Vecef_m/s : Inport  Port=3
  GPS_LLA_rad : Inport  Port=4
  QGC_sensor_reinit : Inport  Port=5
  Vairspeed : Inport  Port=6
  elevator_aileron_rudder_deg : Inport  Port=7
  Bus Creator : BusCreator  Inputs=8
  Constant3 : Constant
  Constant4 : Constant  Value=0.8
  Data Type Conversion{,1..3,5..6,8..11} (10 alike) : DataTypeConversion  OutDataTypeStr=single  SaturateOnIntegerOverflow=off  RndMeth=Floor
  Data Type Conversion4 : DataTypeConversion  OutDataTypeStr=uint8  SaturateOnIntegerOverflow=off  RndMeth=Floor
  Data Type Conversion7 : DataTypeConversion  OutDataTypeStr=double  SaturateOnIntegerOverflow=off  RndMeth=Floor
  GPS_Data_Process : Subsystem
  IMU_Data_Process : Subsystem
  Magn_Data_Process : Subsystem
  Mux : Mux  Inputs=3
  QGC_sensor_reinit1 : InportShadow  Port=5
  QGC_sensor_reinit2 : InportShadow  Port=5
  Subsystem : Subsystem
  TOF_Data_Process : Subsystem
  baro_Data_Process : Subsystem
  Sensor_data : Outport
  wires:
  Mux/1 -> Data Type Conversion6/1
  Constant4/1 -> Data Type Conversion9/1
  Constant3/1 -> Data Type Conversion4/1
  Data Type Conversion11/1 -> Bus Creator/8  "elevator_aileron_rudder_deg"
  elevator_aileron_rudder_deg/1 -> Data Type Conversion11/1  "elevator_aileron_rudder_deg"
  Subsystem/1(VairspeedData) -> Bus Creator/6
  Data Type Conversion8/1 -> Subsystem/1(Vairspeed)
  Vairspeed/1 -> Data Type Conversion8/1  "VairspeedData"
  QGC_sensor_reinit/1 -> baro_Data_Process/2(QGC_sensor_reinit), GPS_Data_Process/5(QGC_sensor_reinit)  "QGC_sensor_reinit"
  GPS_Data_Process/1(GPS_Data) -> Bus Creator/2  "GPS_Data"
  IMU_Data_Process/1(IMU_Data) -> Bus Creator/1  "IMU_Data"
  baro_Data_Process/1(BARO_Data) -> Bus Creator/3  "BARO_Data"
  gyro_B_rad/s_ori/1 -> Data Type Conversion/1
  Magn_Data_Process/1(MAGN_Data) -> Bus Creator/4  "MAGN_Data"
  accl_B_m/s_ori/1 -> Data Type Conversion1/1
  GPS_LLA_rad/1 -> Data Type Conversion7/1
  GPS_Vecef_m/s/1 -> Data Type Conversion2/1
  Bus Creator/1 -> Sensor_data/1
  QGC_sensor_reinit1/1 -> Bus Creator/7  "QGC_sensor_reinit"
  TOF_Data_Process/1(TOF_Data) -> Bus Creator/5
  Data Type Conversion/1 -> IMU_Data_Process/1(gyro_B_rad/s_ori)
  Data Type Conversion1/1 -> IMU_Data_Process/2(accl_B_m/s_ori)
  Data Type Conversion2/1 -> GPS_Data_Process/1(GPS_Vecef_m/s)
  Data Type Conversion7/1 -> GPS_Data_Process/2(GPS_LLA_rad)
  Data Type Conversion4/1 -> GPS_Data_Process/3(GPS_fixtype)
  Data Type Conversion9/1 -> GPS_Data_Process/4(hdop_GPS)
  Data Type Conversion5/1 -> baro_Data_Process/1(baro)
  Data Type Conversion6/1 -> Magn_Data_Process/1(magn_B_guass_ori)
  Data Type Conversion10/1 -> TOF_Data_Process/1(TOF_mm_ori)
  Data Type Conversion3/1 -> baro_Data_Process/3(baro_tem)
  QGC_sensor_reinit2/1 -> TOF_Data_Process/2(QGC_sensor_reinit)  "QGC_sensor_reinit"

== system VB_RIFKF_UWB_INS25/No.1_Sensor_Data_Process4 ==
  gyro_B_rad/s_ori : Inport
  accl_B_m/s_ori : Inport  Port=2
  GPS_Vecef_m/s : Inport  Port=3
  GPS_LLA_rad : Inport  Port=4
  QGC_sensor_reinit : Inport  Port=5
  Vairspeed : Inport  Port=6
  elevator_aileron_rudder_deg : Inport  Port=7
  Bus Creator : BusCreator  Inputs=8
  Constant3 : Constant
  Constant4 : Constant  Value=0.8
  Data Type Conversion{,1..3,5..6,8..11} (10 alike) : DataTypeConversion  OutDataTypeStr=single  SaturateOnIntegerOverflow=off  RndMeth=Floor
  Data Type Conversion4 : DataTypeConversion  OutDataTypeStr=uint8  SaturateOnIntegerOverflow=off  RndMeth=Floor
  Data Type Conversion7 : DataTypeConversion  OutDataTypeStr=double  SaturateOnIntegerOverflow=off  RndMeth=Floor
  GPS_Data_Process : Subsystem
  IMU_Data_Process : Subsystem
  Magn_Data_Process : Subsystem
  Mux : Mux  Inputs=3
  QGC_sensor_reinit1 : InportShadow  Port=5
  QGC_sensor_reinit2 : InportShadow  Port=5
  Subsystem : Subsystem
  TOF_Data_Process : Subsystem
  baro_Data_Process : Subsystem
  Sensor_data : Outport
  GPS0 : Outport  Port=2
  GPS1_noerr : Outport  Port=3
  wires:
  GPS_Data_Process/3(GPS_noerr) -> GPS1_noerr/1
  GPS_Data_Process/2(GPS0) -> GPS0/1
  Mux/1 -> Data Type Conversion6/1
  Constant4/1 -> Data Type Conversion9/1
  Constant3/1 -> Data Type Conversion4/1
  Data Type Conversion11/1 -> Bus Creator/8  "elevator_aileron_rudder_deg"
  elevator_aileron_rudder_deg/1 -> Data Type Conversion11/1  "elevator_aileron_rudder_deg"
  Subsystem/1(VairspeedData) -> Bus Creator/6
  Data Type Conversion8/1 -> Subsystem/1(Vairspeed)
  Vairspeed/1 -> Data Type Conversion8/1  "VairspeedData"
  QGC_sensor_reinit/1 -> baro_Data_Process/2(QGC_sensor_reinit), GPS_Data_Process/5(QGC_sensor_reinit)  "QGC_sensor_reinit"
  GPS_Data_Process/1(GPS_Data) -> Bus Creator/2  "GPS_Data"
  IMU_Data_Process/1(IMU_Data) -> Bus Creator/1  "IMU_Data"
  baro_Data_Process/1(BARO_Data) -> Bus Creator/3  "BARO_Data"
  gyro_B_rad/s_ori/1 -> Data Type Conversion/1
  Magn_Data_Process/1(MAGN_Data) -> Bus Creator/4  "MAGN_Data"
  accl_B_m/s_ori/1 -> Data Type Conversion1/1
  GPS_LLA_rad/1 -> Data Type Conversion7/1
  GPS_Vecef_m/s/1 -> Data Type Conversion2/1
  Bus Creator/1 -> Sensor_data/1
  QGC_sensor_reinit1/1 -> Bus Creator/7  "QGC_sensor_reinit"
  TOF_Data_Process/1(TOF_Data) -> Bus Creator/5
  Data Type Conversion/1 -> IMU_Data_Process/1(gyro_B_rad/s_ori)
  Data Type Conversion1/1 -> IMU_Data_Process/2(accl_B_m/s_ori)
  Data Type Conversion2/1 -> GPS_Data_Process/1(GPS_Vecef_m/s)
  Data Type Conversion7/1 -> GPS_Data_Process/2(GPS_LLA_rad)
  Data Type Conversion4/1 -> GPS_Data_Process/3(GPS_fixtype)
  Data Type Conversion9/1 -> GPS_Data_Process/4(hdop_GPS)
  Data Type Conversion5/1 -> baro_Data_Process/1(baro)
  Data Type Conversion6/1 -> Magn_Data_Process/1(magn_B_guass_ori)
  Data Type Conversion10/1 -> TOF_Data_Process/1(TOF_mm_ori)
  Data Type Conversion3/1 -> baro_Data_Process/3(baro_tem)
  QGC_sensor_reinit2/1 -> TOF_Data_Process/2(QGC_sensor_reinit)  "QGC_sensor_reinit"

== system VB_RIFKF_UWB_INS25/Subsystem ==
  SensorData_hf : Inport
  Bus Creator1 : BusCreator  Inputs=6
  Bus Selector : BusSelector  OutputSignals=GPS_Data.pos_N_gps,GPS_Data.pos_E_gps,GPS_Data.pos_D_gps,GPS_Data.vn_gps,GPS_Data.ve_gps,GPS_Data.vd_gps
  SensorData1 : Outport
  wires:
  Bus Selector/4 -> Bus Creator1/4  "<vn_gps>"
  Bus Selector/6 -> Bus Creator1/6  "<vd_gps>"
  Bus Selector/1 -> Bus Creator1/1  "<pos_N_gps>"
  SensorData_hf/1 -> Bus Selector/1
  Bus Creator1/1 -> SensorData1/1  "SensorData1"
  Bus Selector/2 -> Bus Creator1/2  "<pos_E_gps>"
  Bus Selector/3 -> Bus Creator1/3  "<pos_D_gps>"
  Bus Selector/5 -> Bus Creator1/5  "<ve_gps>"

== system VB_RIFKF_UWB_INS25/Subsystem1 ==
  Compare To Constant : simulink/Logic and Bit Operations/Compare To Constant  relop=<=  const=2.1  OutDataTypeStr=boolean
  Compare To Constant1 : simulink/Logic and Bit Operations/Compare To Constant  relop=>=  const=2  OutDataTypeStr=boolean
  Constant5 : Constant  OutDataTypeStr=uint8
  Constant8 : Constant  Value=0  OutDataTypeStr=uint8
  Digital Clock : DigitalClock  SampleTime=dt
  Logical Operator1 : Logic  AllPortsSameDT=off  OutDataTypeStr=boolean
  Switch3 : Switch  Criteria=u2 > Threshold  SaturateOnIntegerOverflow=off  InputSameDT=off
  QGC_sensor_reinit : Outport
  wires:
  Digital Clock/1 -> Compare To Constant1/1, Compare To Constant/1
  Logical Operator1/1 -> Switch3/2
  Constant5/1 -> Switch3/1
  Compare To Constant1/1 -> Logical Operator1/1
  Compare To Constant/1 -> Logical Operator1/2
  Constant8/1 -> Switch3/3
  Switch3/1 -> QGC_sensor_reinit/1

== system VB_RIFKF_UWB_INS25/Subsystem2 ==
  SensorData_zy : Inport
  Bus Creator1 : BusCreator  Inputs=6
  Bus Selector : BusSelector  OutputSignals=GPS_Data.pos_N_gps,GPS_Data.pos_E_gps,GPS_Data.pos_D_gps,GPS_Data.vn_gps,GPS_Data.ve_gps,GPS_Data.vd_gps
  SensorData2 : Outport
  wires:
  Bus Selector/5 -> Bus Creator1/5  "<ve_gps>"
  Bus Selector/3 -> Bus Creator1/3  "<pos_D_gps>"
  Bus Selector/2 -> Bus Creator1/2  "<pos_E_gps>"
  Bus Creator1/1 -> SensorData2/1  "SensorData2"
  SensorData_zy/1 -> Bus Selector/1
  Bus Selector/1 -> Bus Creator1/1  "<pos_N_gps>"
  Bus Selector/6 -> Bus Creator1/6  "<vd_gps>"
  Bus Selector/4 -> Bus Creator1/4  "<vn_gps>"

== system VB_RIFKF_UWB_INS25/Subsystem3 ==
  SensorData_tj : Inport
  Bus Creator1 : BusCreator  Inputs=6
  Bus Selector : BusSelector  OutputSignals=GPS_Data.pos_N_gps,GPS_Data.pos_E_gps,GPS_Data.pos_D_gps,GPS_Data.vn_gps,GPS_Data.ve_gps,GPS_Data.vd_gps
  SensorData3 : Outport
  wires:
  Bus Selector/5 -> Bus Creator1/5  "<ve_gps>"
  Bus Selector/3 -> Bus Creator1/3  "<pos_D_gps>"
  Bus Selector/2 -> Bus Creator1/2  "<pos_E_gps>"
  Bus Creator1/1 -> SensorData3/1  "SensorData2"
  SensorData_tj/1 -> Bus Selector/1
  Bus Selector/1 -> Bus Creator1/1  "<pos_N_gps>"
  Bus Selector/6 -> Bus Creator1/6  "<vd_gps>"
  Bus Selector/4 -> Bus Creator1/4  "<vn_gps>"

== system VB_RIFKF_UWB_INS25/Subsystem4 ==
  Compare To Constant : simulink/Logic and Bit Operations/Compare To Constant  relop=<=  const=2.1  OutDataTypeStr=boolean
  Compare To Constant1 : simulink/Logic and Bit Operations/Compare To Constant  relop=>=  const=2  OutDataTypeStr=boolean
  Constant5 : Constant  OutDataTypeStr=uint8
  Constant8 : Constant  Value=0  OutDataTypeStr=uint8
  Digital Clock : DigitalClock  SampleTime=dt
  Logical Operator1 : Logic  AllPortsSameDT=off  OutDataTypeStr=boolean
  Switch3 : Switch  Criteria=u2 > Threshold  SaturateOnIntegerOverflow=off  InputSameDT=off
  QGC_sensor_reinit : Outport
  wires:
  Switch3/1 -> QGC_sensor_reinit/1
  Constant8/1 -> Switch3/3
  Compare To Constant/1 -> Logical Operator1/2
  Compare To Constant1/1 -> Logical Operator1/1
  Constant5/1 -> Switch3/1
  Logical Operator1/1 -> Switch3/2
  Digital Clock/1 -> Compare To Constant/1, Compare To Constant1/1

== system VB_RIFKF_UWB_INS25/read FC1_hf ==
  Add : Sum  Commented=on
  Bus Creator{,1..4} (5 alike) : BusCreator  Inputs=3
  Constant : Constant  Commented=on  Value=1.7
  Degrees to Radians{,1..4} (5 alike) : simulink_extras/Transformations/Degrees to Radians
  From Workspace1 : FromWorkspace  VariableName=[time(1:(end-1)),FCS1.data_hf_st.Vn(1:(end-1))]
  From Workspace10 : FromWorkspace  VariableName=[time(1:(end-1)),FCS1.data_hf_st.Ve(1:(end-1))]
  From Workspace11 : FromWorkspace  VariableName=[time(1:(end-1)),FCS1.data_hf_st.Vu(1:(end-1))]
  From Workspace12 : FromWorkspace  VariableName=[time(1:(end-1)),FCS1.data_hf_st.gy(1:(end-1))]
  From Workspace13 : FromWorkspace  VariableName=[time(1:(end-1)),FCS1.data_hf_st.gz(1:(end-1))]
  From Workspace14 : FromWorkspace  VariableName=[time(1:(end-1)),FCS1.data_hf_st.Ax(1:(end-1))]
  From Workspace15 : FromWorkspace  VariableName=[time(1:(end-1)),FCS1.data_hf_st.Ay(1:(end-1))]
  From Workspace16 : FromWorkspace  VariableName=[time(1:(end-1)),FCS1.data_hf_st.Az(1:(end-1))]
  From Workspace17 : FromWorkspace  VariableName=[time(1:(end-1)),FCS1.data_hf_st.roll(1:(end-1))]
  From Workspace18 : FromWorkspace  VariableName=[time(1:(end-1)),FCS1.data_hf_st.pitch(1:(end-1))]
  From Workspace19 : FromWorkspace  VariableName=[time(1:(end-1)),FCS1.data_hf_st.yaw(1:(end-1))]
  From Workspace2 : FromWorkspace  VariableName=[time(1:(end-1)),FCS1.data_hf_st.gx(1:(end-1))]
  From Workspace20 : FromWorkspace  VariableName=[time(1:(end-1)),wy_mv(1:(end-1))']
  From Workspace21 : FromWorkspace  VariableName=[time(1:(end-1)),wz_mv(1:(end-1))']
  From Workspace22 : FromWorkspace  VariableName=[time(1:(end-1)),wx_mv(1:(end-1))']
  From Workspace23 : FromWorkspace  VariableName=[time(1:(end-1)),Fy2(1:(end-1))]
  From Workspace24 : FromWorkspace  VariableName=[time(1:(end-1)),Fz2(1:(end-1))]
  From Workspace25 : FromWorkspace  VariableName=[time(1:(end-1)),Fx2(1:(end-1))]
  From Workspace3 : FromWorkspace  Commented=on  VariableName=[All.t',All.Yeast]
  From Workspace4 : FromWorkspace  Commented=on  VariableName=[All.t',All.Xnorth]
  From Workspace5 : FromWorkspace  Commented=on  VariableName=[All.t',All.mh]
  From Workspace6 : FromWorkspace  Commented=on  VariableName=[All.t',All.Vc]
  From Workspace7 : FromWorkspace  VariableName=[time(1:(end-1)),FCS1.data_hf_st.lat(1:(end-1))]
  From Workspace8 : FromWorkspace  VariableName=[time(1:(end-1)),FCS1.data_hf_st.lon(1:(end-1))]
  From Workspace9 : FromWorkspace  VariableName=[time(1:(end-1)),FCS1.data_hf_st.height(1:(end-1))]
  Gain : Gain  Commented=on  Gain=1/3.6
  Gain1 : Gain  Gain=-1
  Gain2 : Gain  Commented=on  Gain=-1
  MATLAB Function : MATLAB Function  TreatAsAtomicUnit=on
  Mux : Mux  Inputs=3
  Mux1 : Mux  Inputs=3
  Mux2 : Mux  Inputs=3
  Scope{,1..2,4..9} (9 alike) : Scope
  Scope3 : Scope  Commented=on
  Subsystem : Subsystem
  Subsystem1 : Subsystem
  Subsystem2 : Subsystem
  Subsystem3 : Subsystem
  Subsystem4 : Subsystem
  Subsystem5 : Subsystem
  Subsystem6 : Subsystem
  Subsystem7 : Subsystem
  Subsystem8 : Subsystem
  vned_GPS : Outport
  Pned_GPS : Outport  Port=2
  Vair : Outport  Port=3
  GPS_lla_rad : Outport  Port=4
  wxyz : Outport  Port=5
  fbxyz : Outport  Port=6
  att_ref : Outport  Port=7
  wxyz_mv : Outport  Port=8
  wxyz_add : Outport  Port=9
  wires:
  Mux/1 -> Scope2/1, vned_GPS/1
  Mux1/1 -> Scope1/1, Pned_GPS/1
  Add/1 -> Vair/1
  Constant/1 -> Add/2
  Degrees to Radians1/1 -> Mux2/2
  Degrees to Radians/1 -> Mux2/1
  From Workspace7/1 -> Degrees to Radians/1  "lat"
  From Workspace8/1 -> Degrees to Radians1/1  "lon"
  Mux2/1 -> GPS_lla_rad/1, Scope/1
  From Workspace9/1 -> Mux2/3  "altitude"
  Gain2/1 -> Mux1/3
  Gain1/1 -> Mux/3
  From Workspace3/1 -> Mux1/2
  From Workspace4/1 -> Mux1/1
  Gain/1 -> Scope3/1, Add/1
  From Workspace6/1 -> Gain/1
  From Workspace1/1 -> Mux/1  "vn"
  From Workspace10/1 -> Mux/2  "ve"
  From Workspace5/1 -> Gain2/1
  From Workspace11/1 -> Gain1/1
  Subsystem/1(y) -> Bus Creator/1
  From Workspace2/1 -> Subsystem/1(u)
  Subsystem1/1(y) -> Bus Creator/2
  From Workspace16/1 -> Bus Creator1/3
  Bus Creator/1 -> Scope4/1, Degrees to Radians2/1
  From Workspace14/1 -> Bus Creator1/1
  From Workspace15/1 -> Bus Creator1/2
  From Workspace12/1 -> Scope7/1, Subsystem1/1(u)
  Degrees to Radians2/1 -> wxyz/1, Scope6/1
  Subsystem2/1(y) -> Bus Creator/3
  From Workspace13/1 -> Subsystem2/1(u)
  Bus Creator1/1 -> fbxyz/1, Scope5/1
  From Workspace19/1 -> MATLAB Function/1(dpsi)
  Bus Creator2/1 -> Scope9/1, att_ref/1, Scope8/1
  From Workspace17/1 -> Bus Creator2/1  "roll"
  From Workspace18/1 -> Bus Creator2/2  "pitch"
  MATLAB Function/1(y) -> Bus Creator2/3  "yaw"
  From Workspace21/1 -> Subsystem5/1(u)
  Subsystem5/1(y) -> Bus Creator3/3
  From Workspace20/1 -> Subsystem4/1(u)
  Subsystem4/1(y) -> Bus Creator3/2
  From Workspace22/1 -> Subsystem3/1(u)
  Subsystem3/1(y) -> Bus Creator3/1
  Bus Creator3/1 -> Degrees to Radians3/1
  Degrees to Radians3/1 -> wxyz_mv/1
  Degrees to Radians4/1 -> wxyz_add/1
  Bus Creator4/1 -> Degrees to Radians4/1
  Subsystem6/1(y) -> Bus Creator4/1
  From Workspace25/1 -> Subsystem6/1(u)
  Subsystem7/1(y) -> Bus Creator4/2
  From Workspace23/1 -> Subsystem7/1(u)
  Subsystem8/1(y) -> Bus Creator4/3
  From Workspace24/1 -> Subsystem8/1(u)
